simulink model "heatex_sim"  (Simulink 7.6)
settings: Solver=ode4  StartTime=0.0  StopTime=200  FixedStep=2  RelTol=1e-3
StartFcn:
  | heatex_clbk('Start')
StopFcn:
  | heatex_clbk('Stop')
libraries: cstblocks x4, simulink x2
CloseFcn:
  | heatex_clbk('Close')
settings Model: Creator=The MathWorks Inc.
settings DataIOCC: SaveOutput=off  SaveTime=off
settings OptimizationCC: BlockReduction=off  BooleanDataType=off  InitFltsAndDblsToZero=on
settings DebuggingCC: SaveWithParameterizedLinksMsg=none  SignalResolutionControl=TryResolveAllWithWarning  SolverPrmCheckMsg=none  MultiTaskDSMMsg=warning  MultiTaskCondExecSysMsg=none  StrictBusMsg=None
settings HardwareCC: TargetUnknown=on
settings RTWCC: IncludeERTFirstTime=on
settings GRTTargetCC: TargetFcnLib=ansi_tfl_tmw.mat

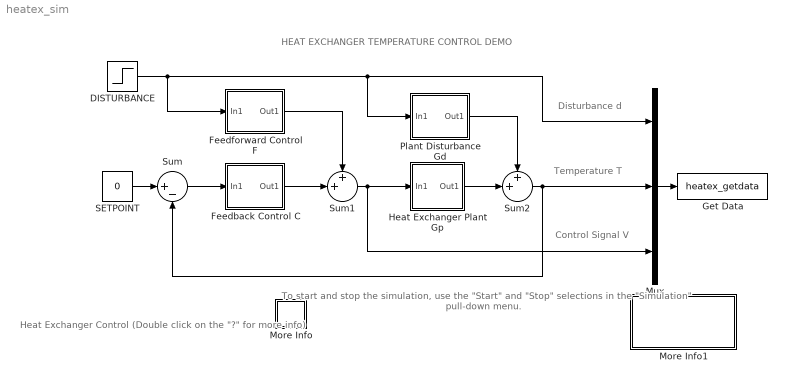
== system heatex_sim ==
  note: HEAT EXCHANGER TEMPERATURE CONTROL DEMO
  note: Control Signal V
  note: Temperature T
  note: Disturbance d
  note: Heat Exchanger Control
      | (Double click on the "?" for more info)
  note: To start and stop the simulation, use the "Start" and
      | "Stop" selections in the "Simulation" pull-down menu.
  DISTURBANCE : Step  Time=20  After=-1  SampleTime=0
  Feedback Control C : Subsystem
  Feedforward Control F : Subsystem
  Get Data : S-Function  FunctionName=heatex_getdata  EnableBusSupport=off
  Heat Exchanger Plant Gp : Subsystem
  More Info : Subsystem
      mask Display: disp('?')
  More Info1 : Subsystem
      settings: OpenFcn=simcad(bdroot);
      mask Display: disp('Double click\nhere for\nSimulink Help')
  Mux : Mux  Inputs=3
  Plant Disturbance Gd : Subsystem
  SETPOINT : Constant  Value=0
  Sum : Sum  Inputs=|+-  SaturateOnIntegerOverflow=on  InputSameDT=on  OutDataTypeStr=Inherit: Same as first input
  Sum1 : Sum  Inputs=++|  SaturateOnIntegerOverflow=on  InputSameDT=on  OutDataTypeStr=Inherit: Same as first input
  Sum2 : Sum  Inputs=++|  SaturateOnIntegerOverflow=on  InputSameDT=on  OutDataTypeStr=Inherit: Same as first input
  wires:
  SETPOINT/1 -> Sum/1
  Sum/1 -> Feedback Control C/1(In1)
  Sum1/1 -> Heat Exchanger Plant Gp/1(In1), Mux/3
  Sum2/1 -> Sum/2, Mux/2
  Mux/1 -> Get Data/1
  Feedforward Control F/1(Out1) -> Sum1/1
  DISTURBANCE/1 -> Feedforward Control F/1(In1), Mux/1, Plant Disturbance Gd/1(In1)
  Feedback Control C/1(Out1) -> Sum1/2
  Heat Exchanger Plant Gp/1(Out1) -> Sum2/2
  Plant Disturbance Gd/1(Out1) -> Sum2/1

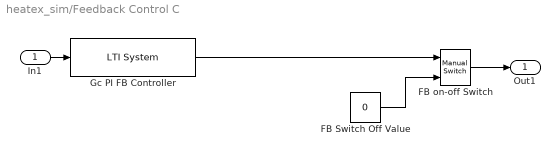
== system heatex_sim/Feedback Control C ==
  In1 : Inport
  FB Switch Off Value : Constant  Value=0
  FB on-off Switch : simulink/Signal Routing/Manual Switch  SystemSampleTime=-1  sw=1  action=0  varsize=off
  Gc PI FB Controller : cstblocks/LTI System  SystemSampleTime=-1  sys=tf([30.31 1.23],[24.56 0])  IC=[]
  Out1 : Outport
  wires:
  In1/1 -> Gc PI FB Controller/1
  Gc PI FB Controller/1 -> FB on-off Switch/1
  FB on-off Switch/1 -> Out1/1
  FB Switch Off Value/1 -> FB on-off Switch/2

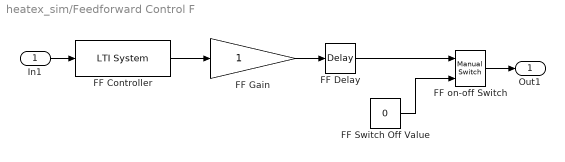
== system heatex_sim/Feedforward Control F ==
  In1 : Inport
  FF Controller : cstblocks/LTI System  SystemSampleTime=-1  sys=tf(-[21.3 1],[25 1])  IC=[]
  FF Delay : TransportDelay  DelayTime=25
      settings: CloseFcn=disp('hello')
  FF Gain : Gain  SaturateOnIntegerOverflow=on  OutDataTypeStr=Inherit: Same as input  ParamDataTypeStr=Inherit: Same as input
      settings: CloseFcn=disp('hello')
  FF Switch Off Value : Constant  Value=0
  FF on-off Switch : simulink/Signal Routing/Manual Switch  SystemSampleTime=-1  sw=0  action=0  varsize=off
  Out1 : Outport
  wires:
  In1/1 -> FF Controller/1
  FF Gain/1 -> FF Delay/1
  FF Controller/1 -> FF Gain/1
  FF Delay/1 -> FF on-off Switch/1
  FF on-off Switch/1 -> Out1/1
  FF Switch Off Value/1 -> FF on-off Switch/2

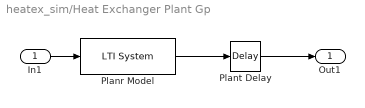
== system heatex_sim/Heat Exchanger Plant Gp ==
  In1 : Inport
  Planr Model : cstblocks/LTI System  SystemSampleTime=-1  sys=tf(1,[21.3 1])  IC=[]
  Plant Delay : TransportDelay  DelayTime=14.7
  Out1 : Outport
  wires:
  In1/1 -> Planr Model/1
  Planr Model/1 -> Plant Delay/1
  Plant Delay/1 -> Out1/1

== system heatex_sim/More Info ==
  note: Try experimenting with switching between
      | using Feedforward and/or Feedback control.
      | Type heatex at the MATLAB prompt to see the demo.
  note: This demonstration shows the temperature control of a continuous stirred
      | tank reactor (CSTR) using a heat exchanger.
      | The controllers have been designed to regulate the temperature of the
      | liquid in the tank when subject to disturbances in the temperature of inlet flow.

== system heatex_sim/More Info1 ==

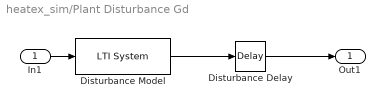
== system heatex_sim/Plant Disturbance Gd ==
  In1 : Inport
  Disturbance Delay : TransportDelay  DelayTime=35
  Disturbance Model : cstblocks/LTI System  SystemSampleTime=-1  sys=tf(1,[25 1])  IC=[]
  Out1 : Outport
  wires:
  Disturbance Delay/1 -> Out1/1
  In1/1 -> Disturbance Model/1
  Disturbance Model/1 -> Disturbance Delay/1
